simulink model "threeTetherGroundStation_th"  (R2018b)
settings: Solver=VariableStepAuto  StartTime=0.0  StopTime=10.0  RelTol=1e-3
values from neighbouring files (symbols this model uses):
  b = 1    [threeTetherGroundStation_ts.m]
  J = 1    [threeTetherGroundStation_ts.m]
  ten1 = [0 1 1]    [threeTetherGroundStation_ts.m]
  ten2 = [0 0 1]    [threeTetherGroundStation_ts.m]
  ten3 = [0 0 1]    [threeTetherGroundStation_ts.m]
libraries: threeTetherGroundStation_cl x1
settings Model: Creator=M.Cobb  LastModifiedBy=mcobb
settings OptimizationCC: BlockReduction=off

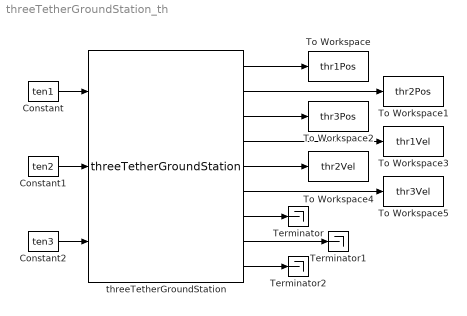
== system threeTetherGroundStation_th ==
  Constant : Constant  Value=ten1
  Constant1 : Constant  Value=ten2
  Constant2 : Constant  Value=ten3
  Terminator : Terminator
  Terminator1 : Terminator
  Terminator2 : Terminator
  To Workspace : ToWorkspace  VariableName=thr1Pos  SaveFormat=Timeseries  SampleTime=-1
  To Workspace1 : ToWorkspace  VariableName=thr2Pos  SaveFormat=Timeseries  SampleTime=-1
  To Workspace2 : ToWorkspace  VariableName=thr3Pos  SaveFormat=Timeseries  SampleTime=-1
  To Workspace3 : ToWorkspace  VariableName=thr1Vel  SaveFormat=Timeseries  SampleTime=-1
  To Workspace4 : ToWorkspace  VariableName=thr2Vel  SaveFormat=Timeseries  SampleTime=-1
  To Workspace5 : ToWorkspace  VariableName=thr3Vel  SaveFormat=Timeseries  SampleTime=-1
  threeTetherGroundStation : threeTetherGroundStation_cl/threeTetherGroundStation  fixed=spinEnable  J=J  b=b  posVec=[0 0 0]  thr1AttachPt=thr1Attach  thr2AttachPt=thr2Attach  thr3AttachPt=thr3Attach  initAngPos=initPos  initAngVel=initVel
  wires:
  Constant/1 -> threeTetherGroundStation/1
  Constant1/1 -> threeTetherGroundStation/2
  Constant2/1 -> threeTetherGroundStation/3
  threeTetherGroundStation/1 -> To Workspace/1
  threeTetherGroundStation/6 -> To Workspace5/1
  threeTetherGroundStation/5 -> To Workspace4/1
  threeTetherGroundStation/4 -> To Workspace3/1
  threeTetherGroundStation/3 -> To Workspace2/1
  threeTetherGroundStation/2 -> To Workspace1/1
  threeTetherGroundStation/7 -> Terminator/1
  threeTetherGroundStation/8 -> Terminator1/1
  threeTetherGroundStation/9 -> Terminator2/1
